simulink model "sim_CAR"  (R2016b)
settings: Solver=FixedStepDiscrete  StartTime=0.0  StopTime=(size(sm_EEG_data,1)-1)/sm.p.EEG.sr  RelTol=1e-3  EnableMultiTasking=on
undefined symbols (not defined in the file): sm
libraries: dspsrcs4 x1
settings Model: Creator=ronens  LastModifiedBy=Csc
settings DataIOCC: LimitDataPoints=on  SaveFormat=Array  SignalLoggingSaveFormat=ModelDataLogs
settings OptimizationCC: ExpressionDepthLimit=2147483647  LifeSpan=inf
settings DebuggingCC: UnderspecifiedInitializationDetection=Classic  MergeDetectMultiDrivingBlocksExec=none  SolverPrmCheckMsg=warning  FcnCallInpInsideContextMsg=warning  StateNameClashWarn=warning  SFUnexpectedBacktrackingDiag=warning  SFNoUnconditionalDefaultTransitionDiag=warning  SFExecutionAtInitializationDiag=none
settings HardwareCC: ProdBitPerPointer=32  ProdBitPerSizeT=32  ProdBitPerPtrDiffT=32  ProdLargestAtomicFloat=None  ProdIntDivRoundTo=Undefined  ProdEndianess=Unspecified  ProdWordSize=32  ProdHWDeviceType=32-bit Generic
settings ModelReferenceCC: PropagateSignalLabelsOutOfModel=off
settings GRTTargetCC: TargetLangStandard=C89/C90 (ANSI)  GeneratePreprocessorConditionals=Disable all
settings ConfigComp: CovMetricSettings=dw  CovHtmlReporting=on  CovSaveCumulativeToWorkspaceVar=on  CovSaveSingleToWorkspaceVar=on  CovExternalEMLEnable=off
settings ConfigurationSet: Description=SimMechanics 2G

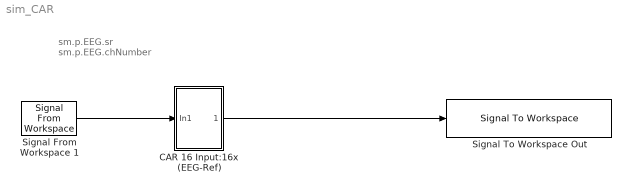
== system sim_CAR ==
  note: sm.p.EEG.sr
      | sm.p.EEG.chNumber
  CAR 16 Input:16x (EEG-Ref) : Subsystem
  Signal From Workspace 1 : dspsrcs4/Signal From Workspace  X=sm_EEG_data  Ts=1/sm.p.EEG.sr  nsamps=1  OutputAfterFinalValue=Setting to zero  ignoreOrWarnInputAndFrameLengths=off  OutputFrames=on
  Signal To Workspace Out : SignalToWorkspace  VariableName=EEG_CAR
      settings: CopyFcn=dspblkcopystw(gcbh);
  wires:
  CAR 16 Input:16x (EEG-Ref)/1(Out1) -> Signal To Workspace Out/1
  Signal From Workspace 1/1 -> CAR 16 Input:16x (EEG-Ref)/1(In1)

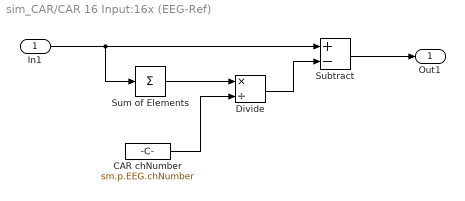
== system sim_CAR/CAR 16 Input:16x (EEG-Ref) ==
  In1 : Inport
  CAR chNumber : Constant  Value=sm.p.EEG.chNumber  VectorParams1D=off  SampleTime=1/sm.p.EEG.sr
  Divide : Product  Inputs=*/
  Subtract : Sum  Inputs=+-
  Sum of Elements : Sum  Inputs=+  InputSameDT=on  OutDataTypeStr=Inherit: Same as first input
  Out1 : Outport
  wires:
  CAR chNumber/1 -> Divide/2
  Sum of Elements/1 -> Divide/1
  In1/1 -> Subtract/1, Sum of Elements/1
  Divide/1 -> Subtract/2
  Subtract/1 -> Out1/1
